simulink model "project"  (R2023a)
settings: Solver=VariableStepAuto  StartTime=0.0  StopTime=10.0  RelTol=1e-3
values from neighbouring files (symbols this model uses):
  b = [0.01 1]    [tfsstwo.m]
  Kd = Kd + 10    (= 20)    [bessaniye.m]    (also in tfss.m = 0.25)
  Ki = 0    [bessaniye.m]    (also in tfss.m = 500)
  Kp = 100    [bessaniye.m]    (also in tfss.m = 21)
undefined symbols (not defined in the file or in its folder): B1, B2, J, J1, J2, K, K1, L, R
libraries: slpidlib x2
settings Model: Creator=monster  LastModifiedBy=monster

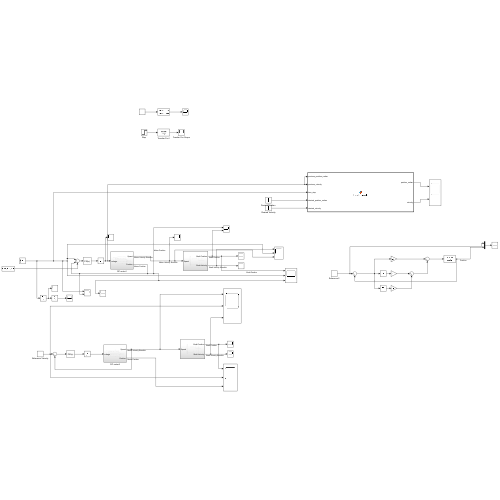
[thumbnail: Simulink's stored preview of the top-level diagram]
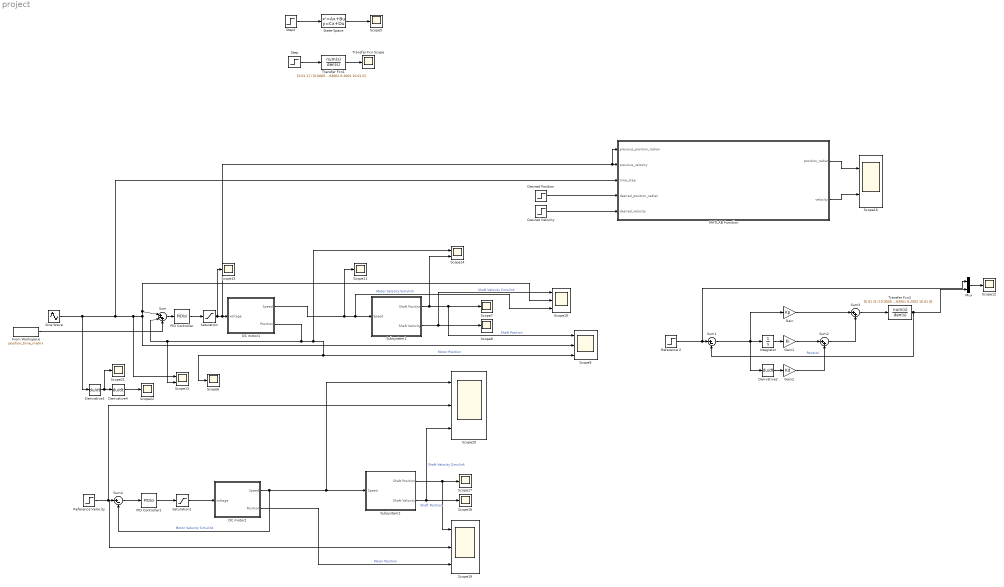
== system project ==
  DC motor1 : Subsystem
  DC motor2 : Subsystem
  Derivative2 : Derivative
  Derivative3 : Derivative
  Derivative4 : Derivative
  "Desired Position " : Step  After=50  SampleTime=0
  Desired Velocity : Step  After=5  SampleTime=0
  From Workspace : FromWorkspace  VariableName=position_time_matrix
  Gain : Gain  Gain=Kp
  Gain1 : Gain  Gain=Ki
  Gain2 : Gain  Gain=Kd
  Integrator : Integrator
  MATLAB Function : MATLAB Function  TreatAsAtomicUnit=on
  Mux : Mux  Inputs=2
  PID Controller : slpidlib/PID Controller  Controller=PID  Form=Parallel  TimeDomain=Continuous-time  UseExternalTs=off  SampleTime=-1  IntegratorMethod=Forward Euler  FilterMethod=Forward Euler  ControllerParametersSource=internal  P=32.545716286284  I=8.52098368694809  UseKiTs=off  D=19.0761370645713  N=387.244472163922  UseFilter=on  TunerSelectOption=Transfer Function Based (PID Tuner App)  InitialConditionSource=internal  InitialConditionForIntegrator=0  InitialConditionForFilter=0  DifferentiatorICPrevScaledInput=0  ExternalReset=none  TrackingMode=off  Kt=1  LimitOutput=off  SatLimitsSource=internal  UpperSaturationLimit=10  LowerSaturationLimit=-10  LinearizeAsGain=on  AntiWindupMode=none  Kb=1  LimitIntegrator=off  UpperIntegratorSaturationLimit=10  LowerIntegratorSaturationLimit=-10  POutMin=[]  POutMax=[]  IOutMin=[]  IOutMax=[]  DOutMin=[]  DOutMax=[]  NOutMin=[]  NOutMax=[]  SumOutMin=[]  SumOutMax=[]  SaturationOutMin=[]  SaturationOutMax=[]  PParamMin=[]  PParamMax=[]  IParamMin=[]  IParamMax=[]  DParamMin=[]  DParamMax=[]  NParamMin=[]  NParamMax=[]  KbParamMin=[]  KbParamMax=[]  KtParamMin=[]  KtParamMax=[]  KbOutMin=[]  KbOutMax=[]  KtOutMin=[]  KtOutMax=[]  IntegratorOutMin=[]  IntegratorOutMax=[]  FilterOutMin=[]  FilterOutMax=[]  SumI1OutMin=[]  SumI1OutMax=[]  SumI2OutMin=[]  SumI2OutMax=[]  SumI3OutMin=[]  SumI3OutMax=[]  SumI4OutMin=[]  SumI4OutMax=[]  SumDOutMin=[]  SumDOutMax=[]  DifferentiatorOutMin=[]  DifferentiatorOutMax=[]  FilterDiffOutCoefMin=[]  FilterDiffOutCoefMax=[]  ReciprocalOutMin=[]  ReciprocalOutMax=[]  SumDenOutMin=[]  SumDenOutMax=[]  SumNumOutMin=[]  SumNumOutMax=[]  DivideOutMin=[]  DivideOutMax=[]  UdiffTsProdOutMin=[]  UdiffTsProdOutMax=[]  NTsProdOutMin=[]  NTsProdOutMax=[]  UintegralTsProdOutMin=[]  UintegralTsProdOutMax=[]  UngainTsProdOutMin=[]  UngainTsProdOutMax=[]  ClampingZeroOutDataTypeStr=Inherit: Inherit via back propagation  ClampingZeroOutMin=[]  ClampingZeroOutMax=[]  FilterDenConstantOutDataTypeStr=Inherit: Inherit via back propagation  FilterDenConstantOutMin=[]  FilterDenConstantOutMax=[]  PCopyOutDataTypeStr=Inherit: Inherit via back propagation  PCopyOutMin=[]  PCopyOutMax=[]  NCopyOutDataTypeStr=Inherit: Inherit via back propagation  NCopyOutMin=[]  NCopyOutMax=[]  IntegratorContinuousStateAttributes=''  IntegratorStateMustResolveToSignalObject=off  IntegratorRTWStateStorageClass=Auto  FilterContinuousStateAttributes=''  FilterStateMustResolveToSignalObject=off  FilterRTWStateStorageClass=Auto  ParallelPVariant=InternalParameters  IdealPVariant=Disabled  IVariant=InternalParameters  DVariant=InternalParameters  IntegratorVariant=Continuous  SatVariant=Disabled  AWVariant=Passthrough  PCopyVariant=Disabled  TRVariant=Disabled  FdbkBlocksVariant=Forward  IdealPFdbkVariant=Disabled  SatFdbkVariant=Disabled  DerivativeFilterVariant=ContFilter  NVariant=InternalParameters  NCopyVariant=Disabled  FilterICVariant=InternalICsFilter  IntegratorICVariant=InternalICs  ExternalResetVariant=Disabled  TRSumVariant=Passthrough  SumFdbkVariant=Disabled  SumVariant=Sum_PID  TsampFilterVariant=InternalTs  TsampNgainVariant=Passthrough  TsampIntegralVariant=Disabled_SignalSpec  ExternalSaturationOutDataTypeStr=Inherit: Same as second input
  PID Controller1 : slpidlib/PID Controller  Controller=PID  Form=Parallel  TimeDomain=Continuous-time  UseExternalTs=off  SampleTime=-1  IntegratorMethod=Forward Euler  FilterMethod=Forward Euler  ControllerParametersSource=internal  P=43.8419795726236  I=12.6968787117754  UseKiTs=off  D=18.6251550360015  N=405.494741877744  UseFilter=on  TunerSelectOption=Transfer Function Based (PID Tuner App)  InitialConditionSource=internal  InitialConditionForIntegrator=0  InitialConditionForFilter=0  DifferentiatorICPrevScaledInput=0  ExternalReset=none  TrackingMode=off  Kt=1  LimitOutput=off  SatLimitsSource=internal  UpperSaturationLimit=10  LowerSaturationLimit=-10  LinearizeAsGain=on  AntiWindupMode=none  Kb=1  LimitIntegrator=off  UpperIntegratorSaturationLimit=10  LowerIntegratorSaturationLimit=-10  POutMin=[]  POutMax=[]  IOutMin=[]  IOutMax=[]  DOutMin=[]  DOutMax=[]  NOutMin=[]  NOutMax=[]  SumOutMin=[]  SumOutMax=[]  SaturationOutMin=[]  SaturationOutMax=[]  PParamMin=[]  PParamMax=[]  IParamMin=[]  IParamMax=[]  DParamMin=[]  DParamMax=[]  NParamMin=[]  NParamMax=[]  KbParamMin=[]  KbParamMax=[]  KtParamMin=[]  KtParamMax=[]  KbOutMin=[]  KbOutMax=[]  KtOutMin=[]  KtOutMax=[]  IntegratorOutMin=[]  IntegratorOutMax=[]  FilterOutMin=[]  FilterOutMax=[]  SumI1OutMin=[]  SumI1OutMax=[]  SumI2OutMin=[]  SumI2OutMax=[]  SumI3OutMin=[]  SumI3OutMax=[]  SumI4OutMin=[]  SumI4OutMax=[]  SumDOutMin=[]  SumDOutMax=[]  DifferentiatorOutMin=[]  DifferentiatorOutMax=[]  FilterDiffOutCoefMin=[]  FilterDiffOutCoefMax=[]  ReciprocalOutMin=[]  ReciprocalOutMax=[]  SumDenOutMin=[]  SumDenOutMax=[]  SumNumOutMin=[]  SumNumOutMax=[]  DivideOutMin=[]  DivideOutMax=[]  UdiffTsProdOutMin=[]  UdiffTsProdOutMax=[]  NTsProdOutMin=[]  NTsProdOutMax=[]  UintegralTsProdOutMin=[]  UintegralTsProdOutMax=[]  UngainTsProdOutMin=[]  UngainTsProdOutMax=[]  ClampingZeroOutDataTypeStr=Inherit: Inherit via back propagation  ClampingZeroOutMin=[]  ClampingZeroOutMax=[]  FilterDenConstantOutDataTypeStr=Inherit: Inherit via back propagation  FilterDenConstantOutMin=[]  FilterDenConstantOutMax=[]  PCopyOutDataTypeStr=Inherit: Inherit via back propagation  PCopyOutMin=[]  PCopyOutMax=[]  NCopyOutDataTypeStr=Inherit: Inherit via back propagation  NCopyOutMin=[]  NCopyOutMax=[]  IntegratorContinuousStateAttributes=''  IntegratorStateMustResolveToSignalObject=off  IntegratorRTWStateStorageClass=Auto  FilterContinuousStateAttributes=''  FilterStateMustResolveToSignalObject=off  FilterRTWStateStorageClass=Auto  ParallelPVariant=InternalParameters  IdealPVariant=Disabled  IVariant=InternalParameters  DVariant=InternalParameters  IntegratorVariant=Continuous  SatVariant=Disabled  AWVariant=Passthrough  PCopyVariant=Disabled  TRVariant=Disabled  FdbkBlocksVariant=Forward  IdealPFdbkVariant=Disabled  SatFdbkVariant=Disabled  DerivativeFilterVariant=ContFilter  NVariant=InternalParameters  NCopyVariant=Disabled  FilterICVariant=InternalICsFilter  IntegratorICVariant=InternalICs  ExternalResetVariant=Disabled  TRSumVariant=Passthrough  SumFdbkVariant=Disabled  SumVariant=Sum_PID  TsampFilterVariant=InternalTs  TsampNgainVariant=Passthrough  TsampIntegralVariant=Disabled_SignalSpec  ExternalSaturationOutDataTypeStr=Inherit: Same as second input
  Reference 2 : Step  SampleTime=0
  Reference Velocity : Step  SampleTime=0
  Saturation : Saturate  UpperLimit=50  LowerLimit=0
  Saturation1 : Saturate  UpperLimit=255  LowerLimit=-255
  Scope{9..10,19..20} (4 alike) : Scope  NumInputPorts=3
  Scope{5..8,11..12,15,17..18,21..22} (11 alike) : Scope
  Scope13 : Scope  NumInputPorts=2
  Scope14 : Scope  NumInputPorts=2
  Scope16 : Scope  NumInputPorts=2
  Sine Wave : Sin  SampleTime=0
  State-Space : StateSpace  A=[-32 -1260 -12400 -20020 0; 1 0 0 0 0; 0 1 0 0 0; 0 0 1 0 0; 0 0 0 1 0]  B=[1; 0; 0; 0; 0]  C=[0 0 0 20 2000]  D=[0]  InitialCondition=[0;0;0;0;0]
  Step : Step  After=5  SampleTime=0
  Step2 : Step  After=5  SampleTime=0
  Subsystem1 : Subsystem
  Subsystem2 : Subsystem
  Sum : Sum  Inputs=|+-+
  Sum1 : Sum  Inputs=|+-
  Sum2 : Sum  Inputs=|++
  Sum3 : Sum  Inputs=|++
  Sum4 : Sum  Inputs=|+-
  Transfer Fcn Scope : Scope
  Transfer Fcn1 : TransferFcn  Numerator=[0.01 1]  Denominator=[0.0005 0.016 0.63001 6.2002 10.01 0]
  Transfer Fcn2 : TransferFcn  Numerator=[0.01 1]  Denominator=[0.0005 0.016 0.63001 6.2002 10.01 0]
  wires:
  From Workspace/1 -> Sum/3
  Integrator/1 -> Gain1/1
  Derivative4/1 -> Scope22/1
  "Desired Position "/1 -> MATLAB Function/4(desired_position_radian)
  DC motor2/1(Speed) -> Scope20/1, Subsystem2/1(Speed), Sum4/2  "Motor Velocity Simulink"
  Gain1/1 -> Sum2/1
  Derivative3/1 -> Scope21/1, Derivative4/1
  MATLAB Function/1(position_radian) -> Scope16/1
  Reference Velocity/1 -> Scope20/2, Scope19/2, Sum4/1
  Sum/1 -> PID Controller/1
  Reference 2/1 -> Mux/1, Sum1/1
  Sum4/1 -> PID Controller1/1
  Subsystem2/2(Shaft Velocity) -> Scope20/3, Scope18/1  "Shaft Velocity Simulink"
  Gain/1 -> Sum3/1
  Transfer Fcn2/1 -> Sum1/2, Mux/2  "Position"
  Subsystem1/2(Shaft Velocity) -> Scope10/1, Scope8/1  "Shaft Velocity Simulink"
  Desired Velocity/1 -> MATLAB Function/5(desired_velocity)
  PID Controller1/1 -> Saturation1/1
  MATLAB Function/2(velocity) -> Scope16/2
  Saturation/1 -> Scope15/1, MATLAB Function/1(previous_position_radian), MATLAB Function/2(previous_velocity), DC motor1/1(voltage)
  Subsystem1/1(Shaft Position) -> Scope14/2, Scope9/1, Scope7/1  "Shaft Position"
  Gain2/1 -> Sum2/2
  Sum2/1 -> Sum3/2
  Derivative2/1 -> Gain2/1
  Subsystem2/1(Shaft Position) -> Scope19/1, Scope17/1  "Shaft Position"
  PID Controller/1 -> Saturation/1
  Sum3/1 -> Transfer Fcn2/1
  Sum1/1 -> Derivative2/1, Gain/1, Integrator/1
  DC motor2/2(Position) -> Scope19/3  "Motor Position"
  Sine Wave/1 -> MATLAB Function/3(time_step), Scope13/1, Scope10/2, Sum/1, Scope9/2, Derivative3/1
  DC motor1/1(Speed) -> Scope11/1, Scope10/3, Subsystem1/1(Speed)  "Motor Velocity Simulink"
  Mux/1 -> Scope12/1
  Saturation1/1 -> DC motor2/1(voltage)
  DC motor1/2(Position) -> Scope13/2, Sum/2, Scope6/1, Scope9/3, Scope14/1  "Motor Position"
  State-Space/1 -> Scope5/1
  Step2/1 -> State-Space/1
  Step/1 -> Transfer Fcn1/1
  Transfer Fcn1/1 -> Transfer Fcn Scope/1

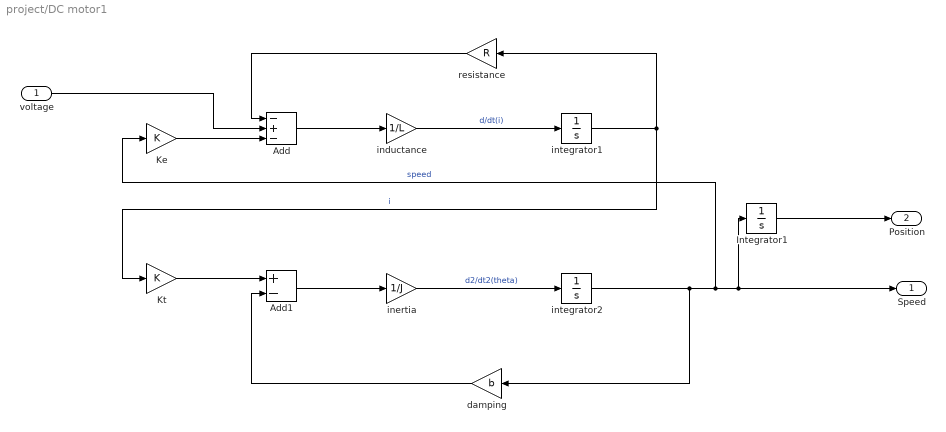
== system project/DC motor1 ==
  voltage : Inport
  Add : Sum  Inputs=-+-
  Add1 : Sum  Inputs=+-
  Integrator1 : Integrator
  Ke : Gain  Gain=K
  Kt : Gain  Gain=K
  damping : Gain  Gain=b
  "inductance " : Gain  Gain=1/L
  inertia : Gain  Gain=1/J
  integrator1 : Integrator
  integrator2 : Integrator
  resistance : Gain  Gain=R
  Speed : Outport
  Position : Outport  Port=2
  wires:
  damping/1 -> Add1/2
  Add1/1 -> inertia/1
  Kt/1 -> Add1/1
  integrator1/1 -> resistance/1, Kt/1  "i"
  Add/1 -> "inductance "/1
  voltage/1 -> Add/2
  resistance/1 -> Add/1
  inertia/1 -> integrator2/1  "d2/dt2(theta)"
  integrator2/1 -> damping/1, Integrator1/1, Speed/1, Ke/1  "speed"
  Ke/1 -> Add/3
  "inductance "/1 -> integrator1/1  "d/dt(i)"
  Integrator1/1 -> Position/1

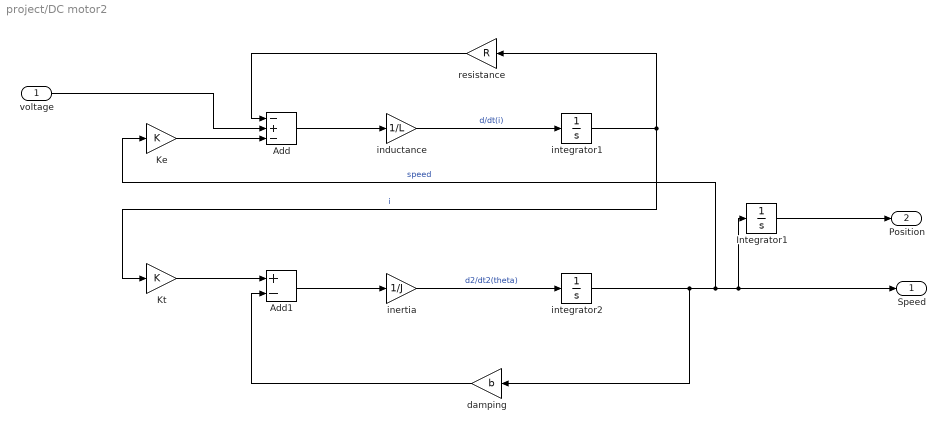
== system project/DC motor2 ==
  voltage : Inport
  Add : Sum  Inputs=-+-
  Add1 : Sum  Inputs=+-
  Integrator1 : Integrator
  Ke : Gain  Gain=K
  Kt : Gain  Gain=K
  damping : Gain  Gain=b
  "inductance " : Gain  Gain=1/L
  inertia : Gain  Gain=1/J
  integrator1 : Integrator
  integrator2 : Integrator
  resistance : Gain  Gain=R
  Speed : Outport
  Position : Outport  Port=2
  wires:
  damping/1 -> Add1/2
  Add1/1 -> inertia/1
  Kt/1 -> Add1/1
  integrator1/1 -> resistance/1, Kt/1  "i"
  Add/1 -> "inductance "/1
  voltage/1 -> Add/2
  resistance/1 -> Add/1
  inertia/1 -> integrator2/1  "d2/dt2(theta)"
  integrator2/1 -> damping/1, Integrator1/1, Speed/1, Ke/1  "speed"
  Ke/1 -> Add/3
  "inductance "/1 -> integrator1/1  "d/dt(i)"
  Integrator1/1 -> Position/1

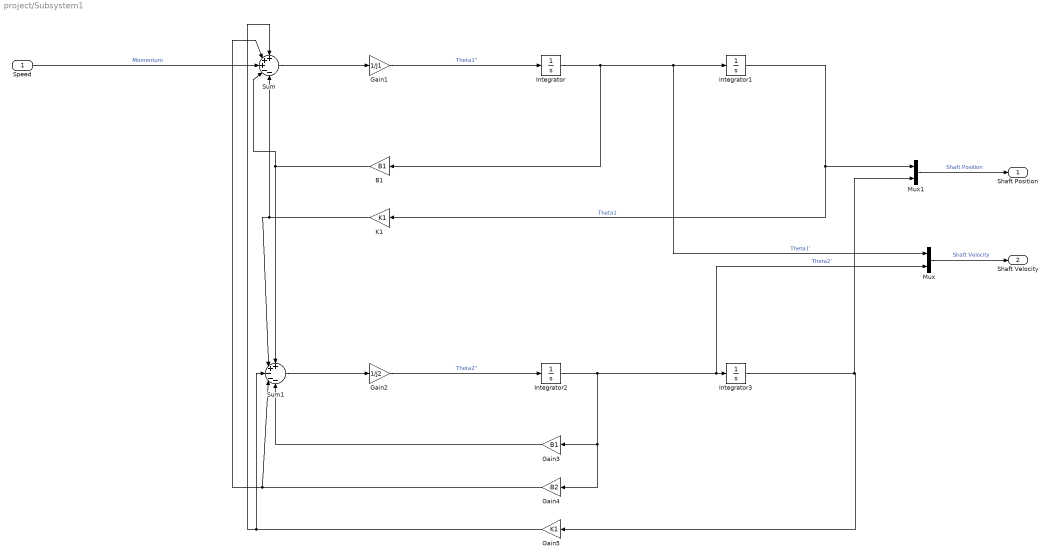
== system project/Subsystem1 ==
  Speed : Inport
  B1 : Gain  Gain=B1
  Gain1 : Gain  Gain=1/J1
  Gain2 : Gain  Gain=1/J2
  Gain3 : Gain  Gain=B1
  Gain4 : Gain  Gain=B2
  Gain5 : Gain  Gain=K1
  Integrator{,1..3} (4 alike) : Integrator
  K1 : Gain  Gain=K1
  Mux : Mux  Inputs=2
  Mux1 : Mux  Inputs=2
  Sum : Sum  Inputs=+++--
  Sum1 : Sum  Inputs=++---
  Shaft Position : Outport
  Shaft Velocity : Outport  Port=2
  wires:
  Gain5/1 -> Sum1/3, Sum/1
  Integrator3/1 -> Gain5/1, Mux1/2
  Gain4/1 -> Sum/2, Sum1/4
  Gain3/1 -> Sum1/5
  Integrator2/1 -> Mux/2, Integrator3/1, Gain3/1, Gain4/1  "Theta2'"
  Gain2/1 -> Integrator2/1  "Theta2''"
  Sum1/1 -> Gain2/1
  K1/1 -> Sum1/2, Sum/5
  Integrator1/1 -> Mux1/1, K1/1  "Theta1"
  B1/1 -> Sum/4, Sum1/1
  Integrator/1 -> Mux/1, Integrator1/1, B1/1  "Theta1'"
  Gain1/1 -> Integrator/1  "Theta1''"
  Speed/1 -> Sum/3  "Momentum"
  Sum/1 -> Gain1/1
  Mux1/1 -> Shaft Position/1  "Shaft Position"
  Mux/1 -> Shaft Velocity/1  "Shaft Velocity"

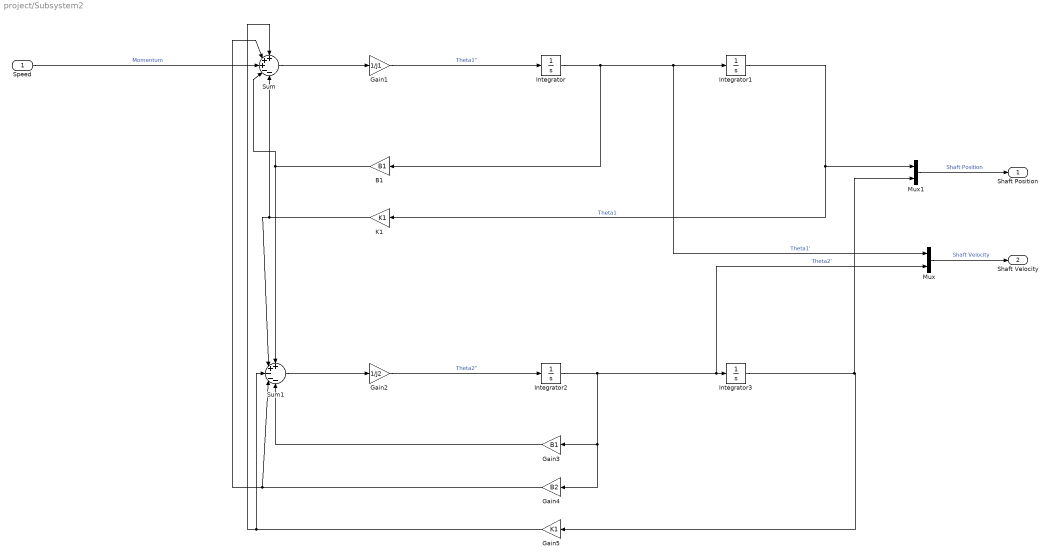
== system project/Subsystem2 ==
  Speed : Inport
  B1 : Gain  Gain=B1
  Gain1 : Gain  Gain=1/J1
  Gain2 : Gain  Gain=1/J2
  Gain3 : Gain  Gain=B1
  Gain4 : Gain  Gain=B2
  Gain5 : Gain  Gain=K1
  Integrator{,1..3} (4 alike) : Integrator
  K1 : Gain  Gain=K1
  Mux : Mux  Inputs=2
  Mux1 : Mux  Inputs=2
  Sum : Sum  Inputs=+++--
  Sum1 : Sum  Inputs=++---
  Shaft Position : Outport
  Shaft Velocity : Outport  Port=2
  wires:
  Gain5/1 -> Sum1/3, Sum/1
  Integrator3/1 -> Gain5/1, Mux1/2
  Gain4/1 -> Sum/2, Sum1/4
  Gain3/1 -> Sum1/5
  Integrator2/1 -> Mux/2, Integrator3/1, Gain3/1, Gain4/1  "Theta2'"
  Gain2/1 -> Integrator2/1  "Theta2''"
  Sum1/1 -> Gain2/1
  K1/1 -> Sum1/2, Sum/5
  Integrator1/1 -> Mux1/1, K1/1  "Theta1"
  B1/1 -> Sum/4, Sum1/1
  Integrator/1 -> Mux/1, Integrator1/1, B1/1  "Theta1'"
  Gain1/1 -> Integrator/1  "Theta1''"
  Speed/1 -> Sum/3  "Momentum"
  Sum/1 -> Gain1/1
  Mux1/1 -> Shaft Position/1  "Shaft Position"
  Mux/1 -> Shaft Velocity/1  "Shaft Velocity"

== matlab function project/MATLAB Function ==
  data: previous_position_radian input; position_radian output; previous_velocity input; time_step input; desired_position_radian input; desired_velocity input; velocity output
function [position_radian, velocity] = simulate_encoder(previous_position_radian, previous_velocity, time_step, desired_position_radian, desired_velocity)
    % Simülasyon parametreleri
    encoder_resolution = 1000; % Kodlayıcı çözünürlüğü (pulse/sayı)
    max_velocity = 10; % Maksimum hız (rad/s)

    % Pozisyonun radyan cinsinden hesaplanması
    previous_position_pulse = previous_position_radian * encoder_resolution / (2 * pi);

    % Hız kontrolü: Motorun istenen hıza ulaşması
    if desired_position_radian > previous_position_radian
        motor_velocity = min(desired_velocity, max_velocity); % İleri hareket için
    else
        motor_velocity = max(-desired_velocity, -max_velocity); % Geri hareket için
    end

    % Motorun yeni pozisyonu ve hızı
    position_pulse = previous_position_pulse + previous_velocity * time_step;
    velocity = motor_velocity;

    % Kodlayıcı sinyallerinin simülasyonu
    encoder_pulse = motor_velocity / (2 * pi) * encoder_resolution; % Kodlayıcı sinyali (pulse/s)
    position_pulse = mod(position_pulse + encoder_pulse, encoder_resolution); % Pozisyon döngüsü

    % Pozisyonun 0 ile encoder_resolution arasında tutulması
    if position_pulse < 0
        position_pulse = position_pulse + encoder_resolution;
    end

    % Güncellenmiş pozisyonun radyan cinsinden hesaplanması
    position_radian = position_pulse * (2 * pi) / encoder_resolution;
end
